simulink model "CLNN_exp_3dof_2NN_exp"  (R2024b)
settings: Solver=ode1  StartTime=0.0  StopTime=T_all  FixedStep=T_sample  RelTol=1e-3
values from neighbouring files (symbols this model uses):
  a1 = m1 * lc1^2 + I1 + (m2 + m3) * l1^2    [plant_robot_3DoF_2NN.m]    (also in setting_3dof_2NN.m = 8.9995)
  a2 = I2 + m2 * lc2^2 + m3 * l2^2    [plant_robot_3DoF_2NN.m]    (also in setting_3dof_2NN.m = 8.9989)
  cl_tf = 300    [run_CLNN_3dof_2NN.m]
  cl_tf1 = 0    [run_CLNN_3dof_2NN.m]
  cl_tf2 = 1050    [run_CLNN_3dof_2NN.m]
  hidden_neure_count_q = 50    [run_CLNN_3dof_2NN.m]
  hidden_neure_count_s = 30    [run_CLNN_3dof_2NN.m]
  kq1 = 0.0026    [setting_3dof_2NN.m]
  kq2 = 0.0011    [setting_3dof_2NN.m]
  lamda = 5    [run_CLNN_3dof_2NN.m]
  lamda_cl = 0.2    [run_CLNN_3dof_2NN.m]
  lamda_cl_s = 0.2    [run_CLNN_3dof_2NN.m]
  learn_time = 100    [run_CLNN_3dof_2NN.m]
  M = [0.001 0 0 ... (first row only)    [run_CLNN_3dof_2NN.m]
  N = 3    [setting_3dof_2NN.m]
  output_dimension_q = 1*N    [run_CLNN_3dof_2NN.m]
  output_dimension_s = 1*N    [run_CLNN_3dof_2NN.m]
  qd20 = 0    [run_CLNN_3dof_2NN.m]
  use_Tqr = 0    [run_CLNN_3dof_2NN.m]
libraries: qbmove_library x3, QB_pacer_lib x1
settings Model: Creator=zou'zhi'gang  LastModifiedBy=zouzgang
settings SolverCC: AlgebraicLoopSolver=TrustRegion
settings DebuggingCC: UnconnectedInputMsg=warning  UnconnectedOutputMsg=warning  UnconnectedLineMsg=warning
settings ModelReferenceCC: EnableRefExpFcnMdlSchedulingChecks=on
settings RTWCC: GPUComputeCapability=3.5

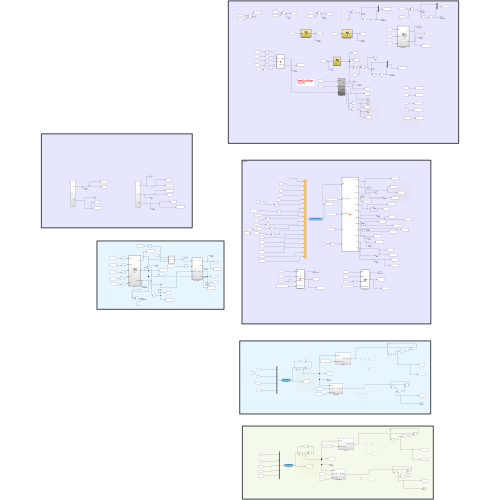
[thumbnail: Simulink's stored preview of the top-level diagram]
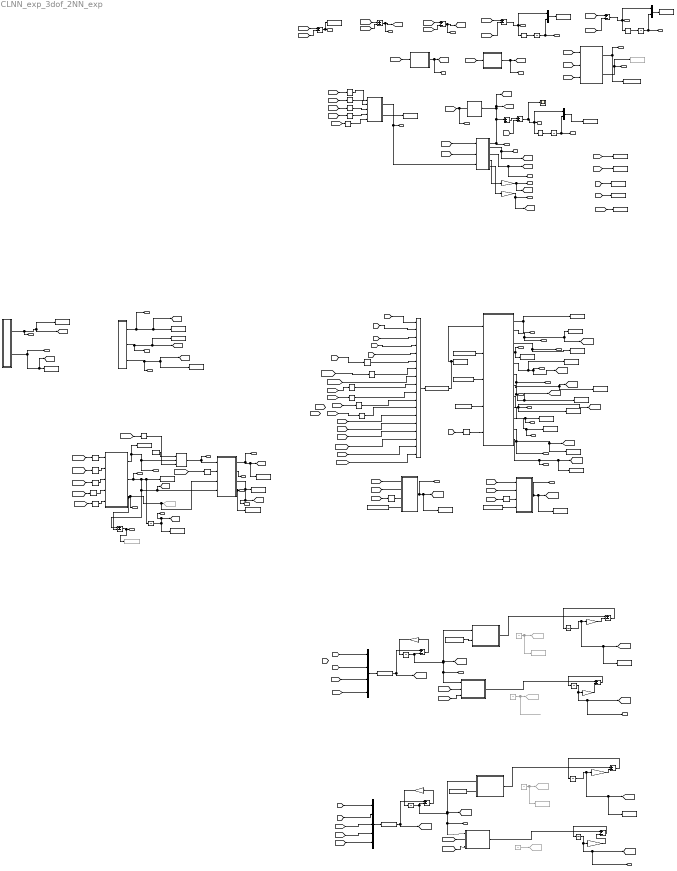
== system CLNN_exp_3dof_2NN_exp ==
  note: 观测器误差
  note: Remember to change the qbmoves IDs and the handle
  Abs1 : Abs  SaturateOnIntegerOverflow=off
  Abs2 : Abs  SaturateOnIntegerOverflow=off
  Abs3 : Abs  SaturateOnIntegerOverflow=off
  Add12 : Sum
  Constant11 : Constant  Value=hidden_neure_count_s
  Constant14 : Constant  Value=N
  Constant16 : Constant  Value=M
  Constant2 : Constant  Value=hidden_neure_count_q
  Constant3 : Constant  Value=hidden_neure_count_s
  Constant4 : Constant  Value=hidden_neure_count_s
  Constant5 : Constant  Value=hidden_neure_count_q
  Constant7 : Constant  Value=hidden_neure_count_q
  Delay{1..21} (21 alike) : Delay  DelayLength=1  InitialCondition=0
  Gain : Gain  Gain=1/265.37
  Gain1 : Gain  Gain=lamda_cl_s
  Gain10 : Gain  Gain=lamda_cl_s
  Gain11 : Gain  Gain=lamda
  Gain12 : Gain  Gain=1/265.37
  Gain2 : Gain  Gain=lamda_cl
  Gain3 : Gain  Gain=lamda_cl
  Gain7 : Gain  Gain=lamda
  Goto3 : Goto  Commented=on  GotoTag=Theta_s
  Goto33 : Goto  Commented=on  GotoTag=Theta_q
  Goto35 : Goto  Commented=on  GotoTag=Theta_W_q
  Goto4 : Goto  Commented=on  GotoTag=Theta_W_s
  Goto83 : Goto  Commented=on  GotoTag=stiff_normal
  Integrator{5..7,12} (4 alike) : Integrator  Commented=on
  Integrator{4,8..9,13..15,17..20} (10 alike) : Integrator
  MATLAB Function : MATLAB Function  TreatAsAtomicUnit=on
  MATLAB Function5 : MATLAB Function  TreatAsAtomicUnit=on
  MATLAB Function6 : MATLAB Function  TreatAsAtomicUnit=on
  Mux1 : Mux  Inputs=[N N N N N]
  Mux2 : Mux  Inputs=[N N N N]
  Mux3 : Mux  Inputs=[N N]
  Mux5 : Mux  Inputs=[N N N N N N N N N N N N N N (hidden_neure_count_q + 1) (hidden_neure_count_q + 1)*output_dimension_q (hidden_neure_count_s + 1) (hidden_neure_count_s + 1)*output_dimension_s]
  Mux7 : Mux  Inputs=[N N]
  Mux8 : Mux  Inputs=[N N]
  Robot : Subsystem
  S-Function4 : S-Function  FunctionName=clnn_control_3dof_2NN  SFunctionDeploymentMode=off  EnableBusSupport=off
  Subsystem4 : Subsystem
  Subtract{1,3..4,6,8,10,14,16..20,22} (13 alike) : Sum  Inputs=+-
  THeta_WW_q : Subsystem
  THeta_WW_s : Subsystem
  Theta error q : MATLAB Function  TreatAsAtomicUnit=on
  Theta error s : MATLAB Function  TreatAsAtomicUnit=on
  Theta_q : Subsystem
  Theta_s : Subsystem
  To Workspace1 : ToWorkspace  VariableName=qd  SampleTime=-1
      settings: Save2DSignal=2-D array (concatenate along first dimension)
  To Workspace10 : ToWorkspace  VariableName=tau_e  SampleTime=-1
      settings: Save2DSignal=2-D array (concatenate along first dimension)
  To Workspace11 : ToWorkspace  VariableName=dqqd  SampleTime=-1
      settings: Save2DSignal=2-D array (concatenate along first dimension)
  To Workspace12 : ToWorkspace  Commented=on  VariableName=Theta_q  SampleTime=-1
      settings: Save2DSignal=2-D array (concatenate along first dimension)
  To Workspace13 : ToWorkspace  VariableName=controlu2  SampleTime=-1
      settings: Save2DSignal=2-D array (concatenate along first dimension)
  To Workspace14 : ToWorkspace  VariableName=controlu1  SampleTime=-1
      settings: Save2DSignal=2-D array (concatenate along first dimension)
  To Workspace15 : ToWorkspace  VariableName=hat_W_q  SampleTime=-1
      settings: Save2DSignal=2-D array (concatenate along first dimension)
  To Workspace16 : ToWorkspace  VariableName=w_un_q_f  SampleTime=-1
      settings: Save2DSignal=2-D array (concatenate along first dimension)
  To Workspace17 : ToWorkspace  Commented=on  VariableName=stiffness1  SampleTime=-1
      settings: Save2DSignal=2-D array (concatenate along first dimension)
  To Workspace18 : ToWorkspace  VariableName=e_S  SampleTime=-1
      settings: Save2DSignal=2-D array (concatenate along first dimension)
  To Workspace19 : ToWorkspace  VariableName=d  SampleTime=-1
      settings: Save2DSignal=2-D array (concatenate along first dimension)
  To Workspace2 : ToWorkspace  VariableName=dqd  SampleTime=-1
      settings: Save2DSignal=2-D array (concatenate along first dimension)
  To Workspace20 : ToWorkspace  VariableName=u_theta1  SampleTime=-1
      settings: Save2DSignal=2-D array (concatenate along first dimension)
  To Workspace21 : ToWorkspace  VariableName=u_theta2  SampleTime=-1
      settings: Save2DSignal=2-D array (concatenate along first dimension)
  To Workspace22 : ToWorkspace  VariableName=e_stiff  SampleTime=-1
      settings: Save2DSignal=2-D array (concatenate along first dimension)
  To Workspace26 : ToWorkspace  VariableName=pd_u  SampleTime=-1
      settings: Save2DSignal=2-D array (concatenate along first dimension)
  To Workspace27 : ToWorkspace  VariableName=model_u  SampleTime=-1
      settings: Save2DSignal=2-D array (concatenate along first dimension)
  To Workspace28 : ToWorkspace  VariableName=Theta_q  SampleTime=-1
      settings: Save2DSignal=2-D array (concatenate along first dimension)
  To Workspace29 : ToWorkspace  Commented=on  VariableName=Theta_s  SampleTime=-1
      settings: Save2DSignal=2-D array (concatenate along first dimension)
  To Workspace30 : ToWorkspace  VariableName=Theta_s  SampleTime=-1
      settings: Save2DSignal=2-D array (concatenate along first dimension)
  To Workspace31 : ToWorkspace  VariableName=Theta_error_s  SampleTime=-1
      settings: Save2DSignal=2-D array (concatenate along first dimension)
  To Workspace33 : ToWorkspace  VariableName=Theta_error_q  SampleTime=-1
      settings: Save2DSignal=2-D array (concatenate along first dimension)
  To Workspace34 : ToWorkspace  VariableName=w_norm_s  SampleTime=-1
      settings: Save2DSignal=2-D array (concatenate along first dimension)
  To Workspace35 : ToWorkspace  VariableName=hat_W_s  SampleTime=-1
      settings: Save2DSignal=2-D array (concatenate along first dimension)
  To Workspace36 : ToWorkspace  VariableName=dstiff  SampleTime=-1
      settings: Save2DSignal=2-D array (concatenate along first dimension)
  To Workspace37 : ToWorkspace  VariableName=dq  SampleTime=-1
      settings: Save2DSignal=2-D array (concatenate along first dimension)
  To Workspace38 : ToWorkspace  VariableName=torque_e  SampleTime=-1
      settings: Save2DSignal=2-D array (concatenate along first dimension)
  To Workspace39 : ToWorkspace  Commented=on  VariableName=stiff_s_nomaic  SampleTime=-1
      settings: Save2DSignal=2-D array (concatenate along first dimension)
  To Workspace4 : ToWorkspace  VariableName=W_V  SampleTime=-1
      settings: Save2DSignal=2-D array (concatenate along first dimension)
  To Workspace40 : ToWorkspace  VariableName=sd  SampleTime=-1
      settings: Save2DSignal=2-D array (concatenate along first dimension)
  To Workspace41 : ToWorkspace  VariableName=stiffness  SampleTime=-1
      settings: Save2DSignal=2-D array (concatenate along first dimension)
  To Workspace42 : ToWorkspace  VariableName=dsd  SampleTime=-1
      settings: Save2DSignal=2-D array (concatenate along first dimension)
  To Workspace43 : ToWorkspace  VariableName=S  SampleTime=-1
      settings: Save2DSignal=2-D array (concatenate along first dimension)
  To Workspace44 : ToWorkspace  VariableName=w_un_s_f  SampleTime=-1
      settings: Save2DSignal=2-D array (concatenate along first dimension)
  To Workspace45 : ToWorkspace  VariableName=tau_e_nomal  SampleTime=-1
      settings: Save2DSignal=2-D array (concatenate along first dimension)
  To Workspace46 : ToWorkspace  VariableName=theta1  SampleTime=-1
      settings: Save2DSignal=2-D array (concatenate along first dimension)
  To Workspace47 : ToWorkspace  VariableName=theta2  SampleTime=-1
      settings: Save2DSignal=2-D array (concatenate along first dimension)
  To Workspace48 : ToWorkspace  VariableName=activation_vec  SampleTime=-1
      settings: Save2DSignal=2-D array (concatenate along first dimension)
  To Workspace49 : ToWorkspace  VariableName=e  SampleTime=-1
      settings: Save2DSignal=2-D array (concatenate along first dimension)
  To Workspace5 : ToWorkspace  VariableName=q  SampleTime=-1
      settings: Save2DSignal=2-D array (concatenate along first dimension)
  To Workspace6 : ToWorkspace  VariableName=w_norm_q  SampleTime=-1
      settings: Save2DSignal=2-D array (concatenate along first dimension)
  To Workspace8 : ToWorkspace  VariableName=epsion  SampleTime=-1
      settings: Save2DSignal=2-D array (concatenate along first dimension)
  To Workspace9 : ToWorkspace  VariableName=w_un_hat  SampleTime=-1
      settings: Save2DSignal=2-D array (concatenate along first dimension)
  Velocity Estimation3 : Subsystem
  Velocity Estimation4 : Subsystem
  Velocity Estimation5 : Subsystem
  phi_3dof_2NN_q : S-Function  FunctionName=phi_3dof_2NN_q  SFunctionDeploymentMode=off  EnableBusSupport=off
  phi_3dof_2NN_s : S-Function  FunctionName=phi_3dof_2NN_s  SFunctionDeploymentMode=off  EnableBusSupport=off
  q-qd : Scope
  s : Subsystem
  stiff and tau1 : Subsystem
  w_un : Subsystem
  w_un_filter : Subsystem  TreatAsAtomicUnit=on
  qd : Outport
  w_un_hat : Outport  Port=2
  WV_q : Outport  Port=3
  epsion : Outport  Port=4
  w_norm : Outport  Port=5
  Theta_error_qq : Outport  Port=6
  controlu1 : Outport  Port=7
  dqd : Outport  Port=8
  dqqd : Outport  Port=9
  tau_e : Outport  Port=10
  w_un_q_f : Outport  Port=11
  phi_filter_q : Outport  Port=12
  controlu2 : Outport  Port=13
  dqq_fq : Outport  Port=14
  u_theta1 : Outport  Port=15
  u_theta2 : Outport  Port=16
  w_q : Outport  Port=17
  model_u : Outport  Port=18
  pd_u : Outport  Port=19
  Theta_W_q : Outport  Port=20
  sd : Outport  Port=21
  dsd : Outport  Port=22
  phi_filter_s : Outport  Port=23
  Theta_W_s : Outport  Port=24
  Theta_error_ss : Outport  Port=25
  w_norm_s : Outport  Port=26
  WV_s : Outport  Port=27
  stiff : Outport  Port=28
  dstiff_nomal : Outport  Port=29
  stiff_s_nomalc : Outport  Port=30
  S : Outport  Port=31
  dS : Outport  Port=32
  w_un_s_f : Outport  Port=33
  dphi1 : Outport  Port=34
  dphi2 : Outport  Port=35
  stiffness1 : Outport  Port=36
  tau_e_nomal1 : Outport  Port=37
  dtheta1 : Outport  Port=38
  dtheta2 : Outport  Port=39
  e : Outport  Port=40
  qe-Integrator : Outport  Port=41
  thtea1 : Outport  Port=42
  theta2 : Outport  Port=43
  q1 : Outport  Port=44
  dq : Outport  Port=45
  activation : Outport  Port=46
  tau1 : Outport  Port=47
  tau2 : Outport  Port=48
  e_S : Outport  Port=49
  e_S-Integrator : Outport  Port=50
  d : Outport  Port=51
  e_stiffness : Outport  Port=52
  e_stiff-Integrator1 : Outport  Port=53
  wires:
  Mux5/1 -> S-Function4/1
  [qd] -> Mux5/1
  [dqd] -> Mux5/2
  [dqqd] -> Mux5/3
  S-Function4/1 -> MATLAB Function6/1(output), To Workspace4/1
  MATLAB Function6/11(W_q) -> WV_q/1, To Workspace15/1, [hat_W_q]
  MATLAB Function6/2(epsion) -> epsion/1, [epsion], To Workspace8/1
  MATLAB Function6/3(w_norm_q) -> To Workspace6/1, w_norm/1
  Integrator6/1 -> To Workspace12/1, Goto33/1
  Integrator7/1 -> Goto35/1
  Integrator8/1 -> Subtract8/2, Theta_q/1(phi_filtter_q), [phi_filter_q], phi_filter_q/1, THeta_WW_q/1(phi_filter)
  Subtract8/1 -> Gain7/1
  Gain7/1 -> Integrator8/1
  [controlu1] -> Mux2/3
  [q] -> Mux2/1
  [controlu2] -> Mux2/4
  Mux2/1 -> phi_3dof_2NN_q/1
  phi_3dof_2NN_q/1 -> [phi_q], Subtract8/1
  [Theta_W_q] -> Theta error q/2(Theta_W_q)
  [Theta_q] -> Theta error q/1(Theta_q)
  Constant7/1 -> Theta error q/4(hidden_neure_count_q)
  Constant5/1 -> Theta_q/2(hidden_neure_count)
  [w_un_q_f] -> THeta_WW_q/2(w_un_q_filter)
  Theta error q/1(Theta_error_q) -> Theta_error_qq/1, To Workspace33/1, [Theta_error_q]
  Constant2/1 -> MATLAB Function6/2(hidden_neure_count_q)
  MATLAB Function6/5(controlu1) -> [controlu1], controlu1/1, To Workspace14/1
  [controlu1] -> Delay1/1
  [controlu2] -> Delay2/1
  Constant14/1 -> MATLAB Function6/4(N)
  MATLAB Function6/1(w_un_hat) -> w_un_hat/1, To Workspace9/1
  Subsystem4/1(qd) -> [qd], To Workspace1/1, qd/1
  Subsystem4/2(dqd) -> To Workspace2/1, [dqd], dqd/1
  Subsystem4/3(dqqd) -> [dqqd], To Workspace11/1, dqqd/1
  w_un/1(tau_e) -> To Workspace10/1, tau_e/1, MATLAB Function/2(tau_e)
  w_un_filter/1(w_un_q_f) -> To Workspace16/1, [w_un_q_f], w_un_q_f/1
  MATLAB Function/1(w_q) -> w_un_filter/1(w_q), w_q/1
  Constant16/1 -> MATLAB Function/1(M)
  MATLAB Function6/6(controlu2) -> To Workspace13/1, [controlu2], controlu2/1
  Delay5/1 -> Theta error q/3(hat_W_vector_q)
  [hat_W_q] -> Delay5/1
  [controlu1] -> Delay6/1
  Delay6/1 -> w_un/1(control_u1)
  [controlu2] -> Delay7/1
  Delay7/1 -> w_un/2(control_u2)
  MATLAB Function6/7(u_theta1) -> u_theta1/1, [u_theta1], To Workspace20/1
  MATLAB Function6/8(u_theta2) -> To Workspace21/1, [u_theta2], u_theta2/1
  [q] -> Delay8/1
  Delay8/1 -> w_un/3(q)
  [q] -> Delay9/1
  [q] -> Delay10/1
  Delay10/1 -> MATLAB Function6/5(q)
  [q] -> Delay12/1
  Delay12/1 -> MATLAB Function/3(q)
  MATLAB Function6/9(pd_u) -> pd_u/1, To Workspace26/1
  MATLAB Function6/10(model_u) -> model_u/1, To Workspace27/1
  Integrator9/1 -> Theta_W_q/1, [Theta_W_q], Gain2/1
  Subtract20/1 -> Integrator15/1
  [dq] -> Mux2/2
  [dq] -> Delay11/1
  THeta_WW_q/1(phi_filter_W_q) -> Subtract10/1
  Gain3/1 -> Subtract20/2
  Integrator15/1 -> Gain3/1, [Theta_q], To Workspace28/1
  Subtract10/1 -> Integrator9/1
  Gain2/1 -> Subtract10/2
  [dq] -> Delay4/1
  Delay11/1 -> w_un_filter/2(dq)
  s/2(Sd) -> sd/1, To Workspace40/1, [sd]
  s/1(dsd) -> dsd/1, To Workspace42/1, [dsd]
  w_un/2(stiff) -> stiff/1, Integrator18/1, To Workspace41/1, [stiffness], w_un_filter/4(stiff), Subtract16/1
  w_un/3(stiff_normal) -> w_un_filter/3(stiff_normal), Goto83/1, dstiff_nomal/1, Subtract16/2
  w_un_filter/2(dqq) -> dqq_fq/1
  w_un_filter/3(w_un_s_f) -> w_un_s_f/1, [w_un_s_f], To Workspace44/1
  [w_un_s_f] -> THeta_WW_q/3(w_un_s_filter)
  Delay1/1 -> Mux5/9
  Delay2/1 -> Mux5/10
  [S] -> Mux5/8
  Delay4/1 -> Mux5/7
  Delay9/1 -> Mux5/6
  [sd] -> Mux5/4
  [dsd] -> Mux5/5
  [w_un_q_f] -> THeta_WW_s/2(w_un_q_filter)
  phi_3dof_2NN_s/1 -> [phi_s], Subtract4/1
  Mux1/1 -> phi_3dof_2NN_s/1
  Gain11/1 -> Integrator13/1
  Integrator12/1 -> Goto4/1
  Constant3/1 -> Theta_s/2(hidden_neure_count)
  [dphi1] -> Mux1/1
  Subtract3/1 -> Integrator4/1
  Integrator14/1 -> Theta_W_s/1, [Theta_W_s], Gain1/1
  Gain10/1 -> Subtract3/2
  [controlu1] -> Mux1/3
  Integrator4/1 -> Gain10/1, [Theta_s], To Workspace30/1
  [w_un_s_f] -> THeta_WW_s/3(w_un_s_filter)
  [dphi2] -> Mux1/2
  [controlu2] -> Mux1/4
  Subtract4/1 -> Gain11/1
  Subtract1/1 -> Integrator14/1
  Integrator13/1 -> Subtract4/2, Theta_s/1(phi_filtter_s), [phi_filter_s], phi_filter_s/1, THeta_WW_s/1(phi_filter)
  Integrator5/1 -> To Workspace29/1, Goto3/1
  Gain1/1 -> Subtract1/2
  Theta error s/1(Theta_error_s) -> Theta_error_ss/1, To Workspace31/1, [Theta_error_s]
  Constant4/1 -> Theta error s/4(hidden_neure_count_s)
  [Theta_s] -> Theta error s/1(Theta_s)
  [Theta_W_s] -> Theta error s/2(Theta_W_s)
  Delay13/1 -> Theta error s/3(hat_W_vector_s)
  [hat_W_s] -> Delay13/1
  Constant11/1 -> MATLAB Function6/3(hidden_neure_count_s)
  MATLAB Function6/4(w_norm_s) -> To Workspace34/1, w_norm_s/1
  MATLAB Function6/12(W_s) -> WV_s/1, To Workspace35/1, [hat_W_s]
  [theta1] -> Delay14/1
  Delay14/1 -> w_un/4(theta1)
  Delay15/1 -> w_un/5(theta2)
  [theta2] -> Delay15/1
  Subtract16/1 -> To Workspace39/1, stiff_s_nomalc/1
  [w_un_q_f] -> Mux5/13
  [w_un_s_f] -> Mux5/14
  [phi_filter_q] -> Mux5/15
  [Theta_error_q] -> Mux5/16
  [phi_filter_s] -> Mux5/17
  [Theta_error_s] -> Mux5/18
  [dtheta1] -> Delay16/1
  [dtheta2] -> Delay17/1
  Delay17/1 -> Mux5/12
  Delay16/1 -> Mux5/11
  w_un_filter/4(dS) -> To Workspace36/1, dS/1
  [dq] -> Mux1/5
  Integrator18/1 -> To Workspace43/1, S/1, [S]
  [q] -> stiff and tau1/3(q)
  [theta1] -> Delay18/1
  [dq] -> To Workspace37/1
  Robot/2(theta1) -> [theta1], thtea1/1
  [q] -> To Workspace5/1
  [torque_e] -> To Workspace38/1
  Velocity Estimation3/1(dtheta1) -> dtheta1/1, [dtheta1]
  stiff and tau1/2(stiff) -> To Workspace17/1, stiffness1/1
  MATLAB Function5/1(activation) -> activation/1, Robot/3(activation)
  Robot/3(theta2) -> theta2/1, [theta2]
  [theta2] -> Delay19/1
  [dtheta2] -> Subtract18/2
  [theta2] -> To Workspace47/1
  Gain/1 -> [tau1], tau1/1
  Gain12/1 -> [tau2], tau2/1
  stiff and tau1/1(tau_e) -> tau_e_nomal1/1, To Workspace45/1
  Robot/1(q) -> q1/1, Velocity Estimation5/1(q), [q], [q_inner], Add12/1
  Subtract14/1 -> q-qd/1, Mux3/1, e/1, Abs1/1
  [theta2] -> stiff and tau1/2(theta2)
  [theta1] -> To Workspace46/1
  [dq] -> Subtract17/1
  Integrator17/1 -> Mux3/2, qe-Integrator/1
  Delay18/1 -> MATLAB Function5/2(theta1)
  Mux3/1 -> To Workspace49/1
  Velocity Estimation4/1(dtheta2) -> dtheta2/1, [dtheta2]
  Robot/4(current1) -> Gain/1
  Delay3/1 -> MATLAB Function5/1(q)
  [theta1] -> stiff and tau1/1(theta1)
  [qd] -> Subtract14/2
  Add12/1 -> Subtract14/1
  [theta2] -> Velocity Estimation4/1(theta2)
  [theta1] -> Velocity Estimation3/1(theta1)
  [dtheta1] -> Subtract17/2
  Delay19/1 -> MATLAB Function5/3(theta2)
  Velocity Estimation5/1(dq) -> dq/1, [dq]
  Robot/5(current2) -> Gain12/1
  Abs1/1 -> Integrator17/1
  [dq] -> Subtract18/1
  [q] -> Delay3/1
  MATLAB Function5/2(activation_vec) -> To Workspace48/1
  Subtract17/1 -> [dphi1], dphi1/1
  Subtract18/1 -> [dphi2], dphi2/1
  Mux7/1 -> To Workspace18/1
  [sd] -> Subtract19/1
  Abs2/1 -> Integrator19/1
  [S] -> Subtract19/2
  Subtract19/1 -> Mux7/1, e_S/1, Abs2/1
  Integrator19/1 -> Mux7/2, e_S-Integrator/1
  [theta2] -> Subtract22/2
  [theta1] -> Subtract22/1
  Subtract22/1 -> To Workspace19/1, d/1
  Subtract6/1 -> Mux8/1, e_stiffness/1, Abs3/1
  [stiffness] -> Subtract6/2
  Integrator20/1 -> Mux8/2, e_stiff-Integrator1/1
  [dsd] -> Subtract6/1
  Abs3/1 -> Integrator20/1
  Mux8/1 -> To Workspace22/1
  Theta_q/1(phi_filter_phi_filte_q) -> Subtract20/1
  Theta_s/1(phi_filter_phi_filter) -> Subtract3/1
  THeta_WW_s/1(phi_filter_W_s) -> Subtract1/1
  [u_theta2] -> Robot/2(u_theta2)
  [u_theta1] -> Robot/1(u_theta1)
  Delay20/1 -> MATLAB Function5/4(u1)
  [u_theta1] -> Delay20/1
  [u_theta2] -> Delay21/1
  Delay21/1 -> MATLAB Function5/5(u2)

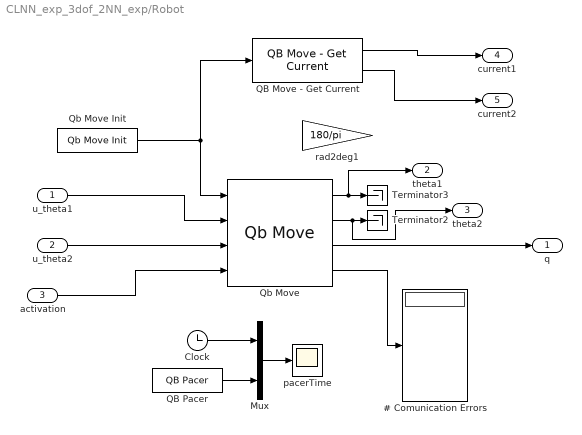
== system CLNN_exp_3dof_2NN_exp/Robot ==
  u_theta1 : Inport
  u_theta2 : Inport  Port=2
  activation : Inport  Port=3
  # Comunication Errors : Display
  Clock : Clock
  Mux : Mux  Inputs=2
  QB Move - Get Current : qbmove_library/QB Move - Get Current  ID=[1,2,3]  CONTROL_MODE=Prime Movers Positions  DAISY_CHAINING=off
      settings: SourceProductName=Qb Move Library
  QB Pacer : QB_pacer_lib/QB Pacer  simTimePerRealTime=1
      settings: SourceProductName=QB Pacer
  Qb Move : qbmove_library/Qb Move  ID=[1,2,3]  ACTIVE_COMM_DIRECTIONS=Both  CONTROL_MODE=Prime Movers Positions  DAISY_CHAINING=off  MAX_ANG=0  SW_LIMIT=inf  OFFSET=0  ACTIVATE=off  WDT=0.0  UNIT=Radians
      settings: SourceProductName=Qb Move Library
  Qb Move Init : qbmove_library/Qb Move Init  NUMBER_OF_COM='COM19'  BAUD_RATE_COM=2000000
      settings: SourceProductName=Qb Move Library
  Terminator2 : Terminator
  Terminator3 : Terminator
  pacerTime : Scope
  rad2deg1 : Gain  Gain=180/pi
  q : Outport
  theta1 : Outport  Port=2
  theta2 : Outport  Port=3
  current1 : Outport  Port=4
  current2 : Outport  Port=5
  wires:
  QB Pacer/1 -> Mux/2
  Clock/1 -> Mux/1
  Qb Move Init/1 -> Qb Move/1, QB Move - Get Current/1
  Mux/1 -> pacerTime/1
  Qb Move/1 -> theta1/1, Terminator3/1
  Qb Move/2 -> theta2/1, Terminator2/1
  u_theta1/1 -> Qb Move/2
  Qb Move/4 -> # Comunication Errors/1
  u_theta2/1 -> Qb Move/3
  Qb Move/3 -> q/1
  activation/1 -> Qb Move/4
  QB Move - Get Current/1 -> current1/1
  QB Move - Get Current/2 -> current2/1

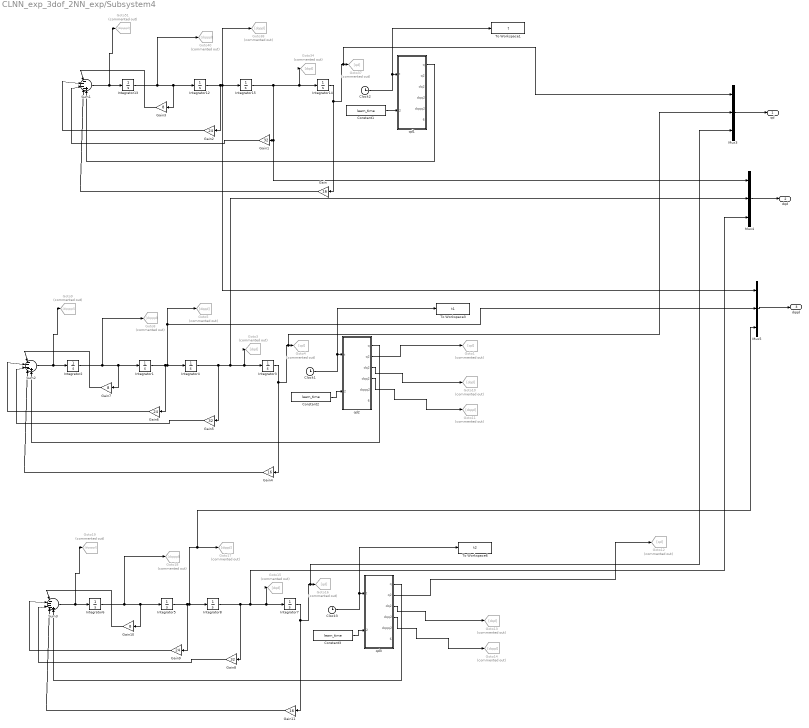
== system CLNN_exp_3dof_2NN_exp/Subsystem4 ==
  Clock1 : Clock
  Clock2 : Clock
  Clock3 : Clock
  Constant1 : Constant  Value=learn_time
  Constant2 : Constant  Value=learn_time
  Constant3 : Constant  Value=learn_time
  Gain : Gain  Gain=16
  Gain1 : Gain  Gain=32
  Gain10 : Gain  Gain=8
  Gain11 : Gain  Gain=16
  Gain2 : Gain  Gain=24
  Gain3 : Gain  Gain=8
  Gain4 : Gain  Gain=16
  Gain5 : Gain  Gain=32
  Gain6 : Gain  Gain=24
  Gain7 : Gain  Gain=8
  Gain8 : Gain  Gain=32
  Gain9 : Gain  Gain=24
  Goto{1,4,12,16,37} (5 alike) : Goto  Commented=on  GotoTag=qd
  Goto{3,10,13,15,34} (5 alike) : Goto  Commented=on  GotoTag=dqd
  Goto{5,11,14,17,38} (5 alike) : Goto  Commented=on  GotoTag=dqqd
  Goto18 : Goto  Commented=on  GotoTag=dqqqd
  Goto19 : Goto  Commented=on  GotoTag=dqqqqd
  Goto40 : Goto  Commented=on  GotoTag=dqqqd
  Goto51 : Goto  Commented=on  GotoTag=dqqqqd
  Goto8 : Goto  Commented=on  GotoTag=dqqqd
  Goto9 : Goto  Commented=on  GotoTag=dqqqqd
  Integrator{1..2,4..8,12..15} (11 alike) : Integrator
  Integrator3 : Integrator  InitialCondition=qd20
  Mux3 : Mux  Inputs=3
  Mux4 : Mux  Inputs=3
  Mux5 : Mux  Inputs=3
  Sum1 : Sum  Inputs=|----+
  Sum2 : Sum  Inputs=|----+
  Sum3 : Sum  Inputs=|----+
  To Workspace1 : ToWorkspace  VariableName=t  SaveFormat=Timeseries  SampleTime=-1
  To Workspace3 : ToWorkspace  VariableName=t1  SaveFormat=Timeseries  SampleTime=-1
  To Workspace6 : ToWorkspace  VariableName=t2  SaveFormat=Timeseries  SampleTime=-1
  qd1 : MATLAB Function  TreatAsAtomicUnit=on
  qd2 : MATLAB Function  TreatAsAtomicUnit=on
  qd3 : MATLAB Function  TreatAsAtomicUnit=on
  qd : Outport
  dqd : Outport  Port=2
  dqqd : Outport  Port=3
  wires:
  Clock2/1 -> To Workspace1/1, qd1/1(t)
  Integrator15/1 -> Mux4/1, Gain1/1, Goto34/1, Integrator14/1
  Integrator13/1 -> Goto40/1, Gain3/1, Integrator12/1
  Sum1/1 -> Goto51/1, Integrator13/1
  Integrator14/1 -> Mux3/1, Goto37/1, Gain/1
  Gain/1 -> Sum1/4
  Integrator12/1 -> Gain2/1, Mux5/1, Goto38/1, Integrator15/1
  Gain2/1 -> Sum1/2
  Gain3/1 -> Sum1/1
  Gain1/1 -> Sum1/3
  qd1/1(q) -> Sum1/5
  Gain5/1 -> Sum2/3
  qd2/1(q) -> Sum2/5
  Gain6/1 -> Sum2/2
  qd2/3(dq2) -> Goto10/1
  Gain7/1 -> Sum2/1
  Integrator1/1 -> Gain6/1, Mux5/2, Goto5/1, Integrator4/1
  qd2/2(q2) -> Goto1/1
  Integrator3/1 -> Mux3/2, Goto4/1, Gain4/1
  qd2/4(dqq2) -> Goto11/1
  Integrator2/1 -> Goto8/1, Gain7/1, Integrator1/1
  Sum2/1 -> Goto9/1, Integrator2/1
  Gain4/1 -> Sum2/4
  Clock1/1 -> To Workspace3/1, qd2/1(t)
  Integrator4/1 -> Gain5/1, Mux4/2, Goto3/1, Integrator3/1
  Integrator7/1 -> Gain11/1, Mux3/3, Goto16/1
  Clock3/1 -> To Workspace6/1, qd3/1(t)
  Integrator8/1 -> Gain8/1, Mux4/3, Goto15/1, Integrator7/1
  Gain10/1 -> Sum3/1
  qd3/2(q2) -> Goto12/1
  qd3/4(dqq2) -> Goto14/1
  Gain8/1 -> Sum3/3
  Sum3/1 -> Goto19/1, Integrator6/1
  Integrator6/1 -> Goto18/1, Gain10/1, Integrator5/1
  Gain9/1 -> Sum3/2
  Gain11/1 -> Sum3/4
  qd3/1(q) -> Sum3/5
  Integrator5/1 -> Gain9/1, Mux5/3, Goto17/1, Integrator8/1
  qd3/3(dq2) -> Goto13/1
  Mux3/1 -> qd/1
  Mux4/1 -> dqd/1
  Mux5/1 -> dqqd/1
  Constant1/1 -> qd1/2(learn_time)
  Constant2/1 -> qd2/2(learn_time)
  Constant3/1 -> qd3/2(learn_time)

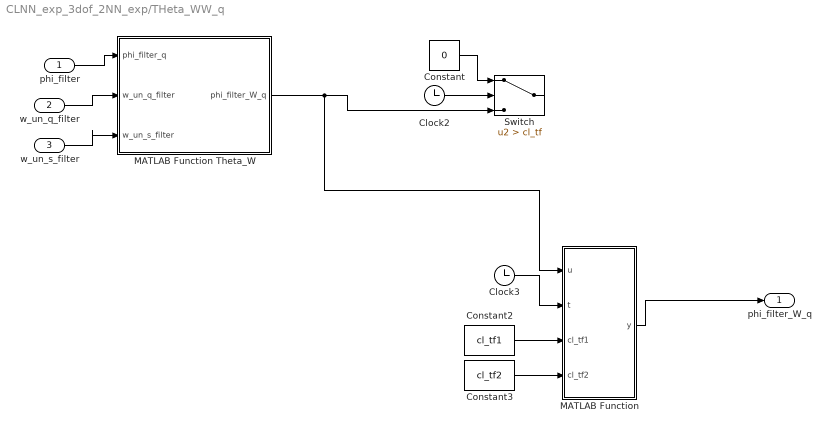
== system CLNN_exp_3dof_2NN_exp/THeta_WW_q ==
  phi_filter : Inport
  w_un_q_filter : Inport  Port=2
  w_un_s_filter : Inport  Port=3
  Clock2 : Clock
  Clock3 : Clock
  Constant : Constant  Value=0
  Constant2 : Constant  Value=cl_tf1
  Constant3 : Constant  Value=cl_tf2
  MATLAB Function : MATLAB Function  TreatAsAtomicUnit=on
  MATLAB Function Theta_W : MATLAB Function  TreatAsAtomicUnit=on
  Switch : Switch  Criteria=u2 > Threshold  Threshold=cl_tf  SaturateOnIntegerOverflow=off  InputSameDT=off
  phi_filter_W_q : Outport
  wires:
  w_un_q_filter/1 -> MATLAB Function Theta_W/2(w_un_q_filter)
  phi_filter/1 -> MATLAB Function Theta_W/1(phi_filter_q)
  Clock2/1 -> Switch/2
  Constant/1 -> Switch/1
  MATLAB Function/1(y) -> phi_filter_W_q/1
  Constant3/1 -> MATLAB Function/4(cl_tf2)
  Clock3/1 -> MATLAB Function/2(t)
  Constant2/1 -> MATLAB Function/3(cl_tf1)
  MATLAB Function Theta_W/1(phi_filter_W_q) -> MATLAB Function/1(u), Switch/3
  w_un_s_filter/1 -> MATLAB Function Theta_W/3(w_un_s_filter)

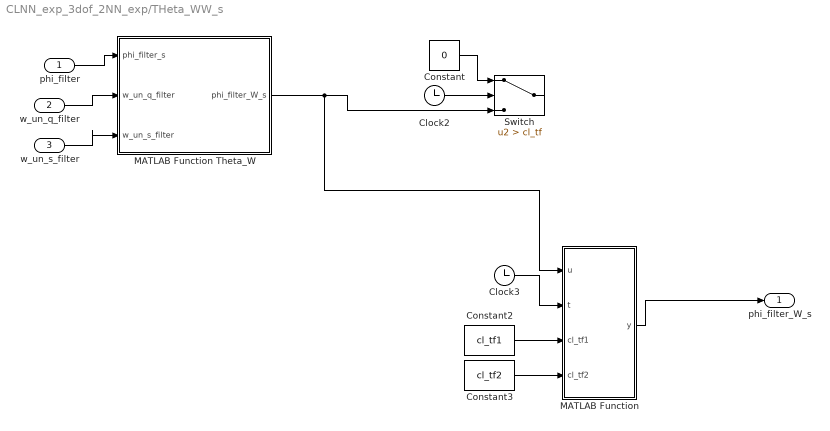
== system CLNN_exp_3dof_2NN_exp/THeta_WW_s ==
  phi_filter : Inport
  w_un_q_filter : Inport  Port=2
  w_un_s_filter : Inport  Port=3
  Clock2 : Clock
  Clock3 : Clock
  Constant : Constant  Value=0
  Constant2 : Constant  Value=cl_tf1
  Constant3 : Constant  Value=cl_tf2
  MATLAB Function : MATLAB Function  TreatAsAtomicUnit=on
  MATLAB Function Theta_W : MATLAB Function  TreatAsAtomicUnit=on
  Switch : Switch  Criteria=u2 > Threshold  Threshold=cl_tf  SaturateOnIntegerOverflow=off  InputSameDT=off
  phi_filter_W_s : Outport
  wires:
  w_un_q_filter/1 -> MATLAB Function Theta_W/2(w_un_q_filter)
  phi_filter/1 -> MATLAB Function Theta_W/1(phi_filter_s)
  Clock2/1 -> Switch/2
  Constant/1 -> Switch/1
  MATLAB Function/1(y) -> phi_filter_W_s/1
  Constant3/1 -> MATLAB Function/4(cl_tf2)
  Clock3/1 -> MATLAB Function/2(t)
  Constant2/1 -> MATLAB Function/3(cl_tf1)
  MATLAB Function Theta_W/1(phi_filter_W_s) -> MATLAB Function/1(u), Switch/3
  w_un_s_filter/1 -> MATLAB Function Theta_W/3(w_un_s_filter)

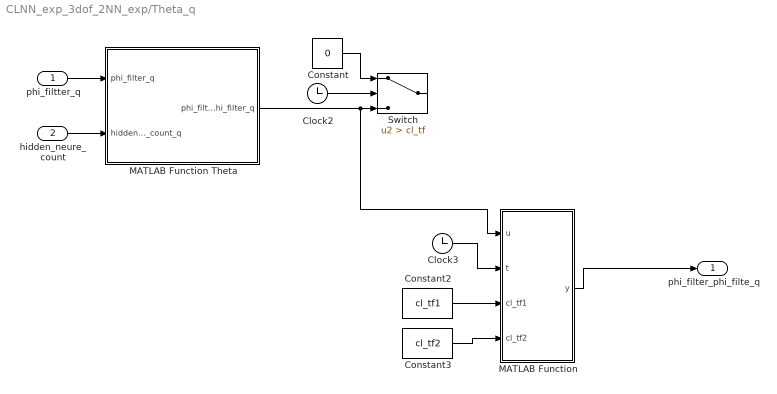
== system CLNN_exp_3dof_2NN_exp/Theta_q ==
  phi_filtter_q : Inport
  hidden_neure_count : Inport  Port=2
  Clock2 : Clock
  Clock3 : Clock
  Constant : Constant  Value=0
  Constant2 : Constant  Value=cl_tf1
  Constant3 : Constant  Value=cl_tf2
  MATLAB Function : MATLAB Function  TreatAsAtomicUnit=on
  MATLAB Function Theta : MATLAB Function  TreatAsAtomicUnit=on
  Switch : Switch  Criteria=u2 > Threshold  Threshold=cl_tf  SaturateOnIntegerOverflow=off  InputSameDT=off
  phi_filter_phi_filte_q : Outport
  wires:
  phi_filtter_q/1 -> MATLAB Function Theta/1(phi_filter_q)
  hidden_neure_count/1 -> MATLAB Function Theta/2(hidden_neure_count_q)
  Clock2/1 -> Switch/2
  Constant/1 -> Switch/1
  MATLAB Function/1(y) -> phi_filter_phi_filte_q/1
  Constant2/1 -> MATLAB Function/3(cl_tf1)
  Constant3/1 -> MATLAB Function/4(cl_tf2)
  MATLAB Function Theta/1(phi_filter_phi_filter_q) -> MATLAB Function/1(u), Switch/3
  Clock3/1 -> MATLAB Function/2(t)

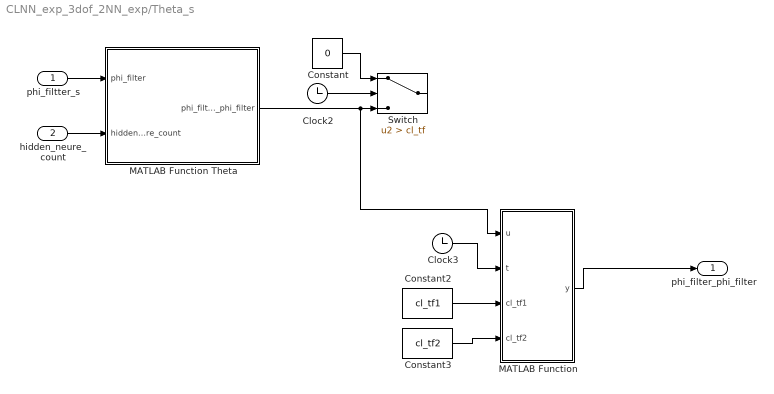
== system CLNN_exp_3dof_2NN_exp/Theta_s ==
  phi_filtter_s : Inport
  hidden_neure_count : Inport  Port=2
  Clock2 : Clock
  Clock3 : Clock
  Constant : Constant  Value=0
  Constant2 : Constant  Value=cl_tf1
  Constant3 : Constant  Value=cl_tf2
  MATLAB Function : MATLAB Function  TreatAsAtomicUnit=on
  MATLAB Function Theta : MATLAB Function  TreatAsAtomicUnit=on
  Switch : Switch  Criteria=u2 > Threshold  Threshold=cl_tf  SaturateOnIntegerOverflow=off  InputSameDT=off
  phi_filter_phi_filter : Outport
  wires:
  phi_filtter_s/1 -> MATLAB Function Theta/1(phi_filter)
  hidden_neure_count/1 -> MATLAB Function Theta/2(hidden_neure_count)
  Clock2/1 -> Switch/2
  Constant/1 -> Switch/1
  MATLAB Function/1(y) -> phi_filter_phi_filter/1
  Constant2/1 -> MATLAB Function/3(cl_tf1)
  Constant3/1 -> MATLAB Function/4(cl_tf2)
  MATLAB Function Theta/1(phi_filter_phi_filter) -> MATLAB Function/1(u), Switch/3
  Clock3/1 -> MATLAB Function/2(t)

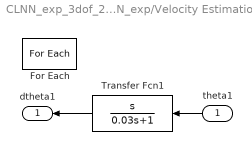
== system CLNN_exp_3dof_2NN_exp/Velocity Estimation3 ==
  theta1 : Inport  Partition=on  PartitionDimension=1  PartitionWidth=1  PartitionOffset=0
  For Each : ForEach  DisableCoverage=on
  Transfer Fcn1 : TransferFcn  Numerator=[1 0]  Denominator=[0.03 1]
  dtheta1 : Outport  ConcatenationDimension=1
  wires:
  theta1/1 -> Transfer Fcn1/1
  Transfer Fcn1/1 -> dtheta1/1

== system CLNN_exp_3dof_2NN_exp/Velocity Estimation4 ==
  theta2 : Inport  Partition=on  PartitionDimension=1  PartitionWidth=1  PartitionOffset=0
  For Each : ForEach  DisableCoverage=on
  Transfer Fcn1 : TransferFcn  Numerator=[1 0]  Denominator=[0.03 1]
  dtheta2 : Outport  ConcatenationDimension=1
  wires:
  theta2/1 -> Transfer Fcn1/1
  Transfer Fcn1/1 -> dtheta2/1

== system CLNN_exp_3dof_2NN_exp/Velocity Estimation5 ==
  q : Inport  Partition=on  PartitionDimension=1  PartitionWidth=1  PartitionOffset=0
  For Each : ForEach  DisableCoverage=on
  Transfer Fcn1 : TransferFcn  Numerator=[1 0]  Denominator=[0.03 1]
  dq : Outport  ConcatenationDimension=1
  wires:
  q/1 -> Transfer Fcn1/1
  Transfer Fcn1/1 -> dq/1

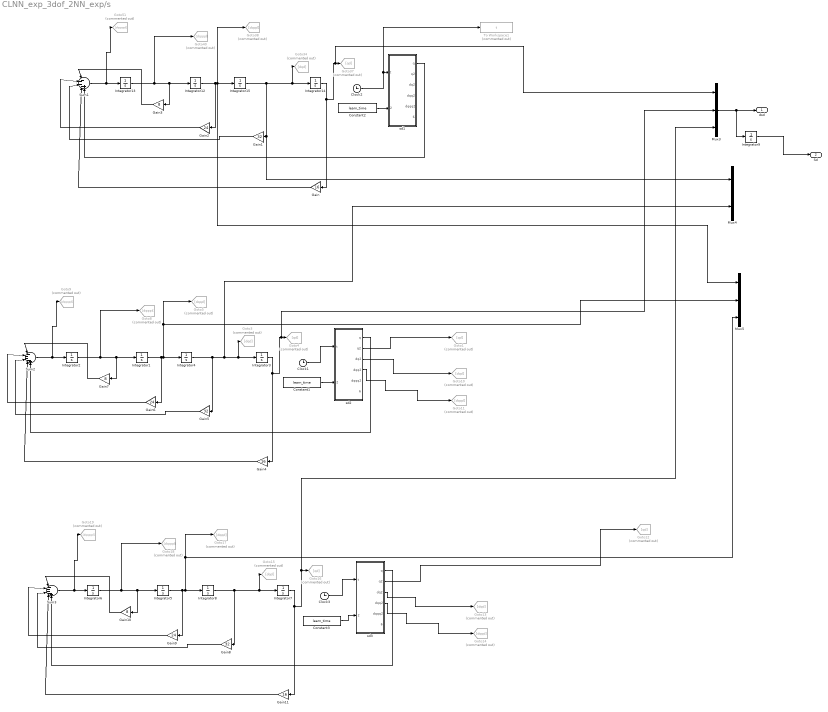
== system CLNN_exp_3dof_2NN_exp/s ==
  Clock1 : Clock
  Clock2 : Clock
  Clock3 : Clock
  Constant1 : Constant  Value=learn_time
  Constant2 : Constant  Value=learn_time
  Constant3 : Constant  Value=learn_time
  Gain : Gain  Gain=16
  Gain1 : Gain  Gain=32
  Gain10 : Gain  Gain=8
  Gain11 : Gain  Gain=16
  Gain2 : Gain  Gain=24
  Gain3 : Gain  Gain=8
  Gain4 : Gain  Gain=16
  Gain5 : Gain  Gain=32
  Gain6 : Gain  Gain=24
  Gain7 : Gain  Gain=8
  Gain8 : Gain  Gain=32
  Gain9 : Gain  Gain=24
  Goto{1,4,12,16,37} (5 alike) : Goto  Commented=on  GotoTag=qd
  Goto{3,10,13,15,34} (5 alike) : Goto  Commented=on  GotoTag=dqd
  Goto{5,11,14,17,38} (5 alike) : Goto  Commented=on  GotoTag=dqqd
  Goto18 : Goto  Commented=on  GotoTag=dqqqd
  Goto19 : Goto  Commented=on  GotoTag=dqqqqd
  Goto40 : Goto  Commented=on  GotoTag=dqqqd
  Goto51 : Goto  Commented=on  GotoTag=dqqqqd
  Goto8 : Goto  Commented=on  GotoTag=dqqqd
  Goto9 : Goto  Commented=on  GotoTag=dqqqqd
  Integrator{1..8,12..13,15} (11 alike) : Integrator
  Integrator14 : Integrator  InitialCondition=0.0333
  Integrator9 : Integrator  InitialCondition=0.0333
  Mux3 : Mux  Inputs=3
  Mux4 : Mux  Inputs=2
  Mux5 : Mux  Inputs=3
  Sum1 : Sum  Inputs=|----+
  Sum2 : Sum  Inputs=|----+
  Sum3 : Sum  Inputs=|----+
  To Workspace1 : ToWorkspace  Commented=on  VariableName=t  SaveFormat=Timeseries  SampleTime=-1
  sd1 : MATLAB Function  TreatAsAtomicUnit=on
  sd2 : MATLAB Function  TreatAsAtomicUnit=on
  sd3 : MATLAB Function  TreatAsAtomicUnit=on
  dsd : Outport
  Sd : Outport  Port=2
  wires:
  Clock2/1 -> To Workspace1/1, sd1/1(t)
  Integrator15/1 -> Mux4/1, Gain1/1, Goto34/1, Integrator14/1
  Integrator13/1 -> Goto40/1, Gain3/1, Integrator12/1
  Sum1/1 -> Goto51/1, Integrator13/1
  Integrator14/1 -> Mux3/1, Goto37/1, Gain/1
  Gain/1 -> Sum1/4
  Integrator12/1 -> Gain2/1, Mux5/1, Goto38/1, Integrator15/1
  Gain2/1 -> Sum1/2
  Gain3/1 -> Sum1/1
  Gain1/1 -> Sum1/3
  sd1/1(q) -> Sum1/5
  Gain5/1 -> Sum2/3
  sd2/1(q) -> Sum2/5
  Gain6/1 -> Sum2/2
  sd2/3(dq2) -> Goto10/1
  Gain7/1 -> Sum2/1
  Integrator1/1 -> Gain6/1, Mux5/2, Goto5/1, Integrator4/1
  sd2/2(q2) -> Goto1/1
  Integrator3/1 -> Mux3/2, Goto4/1, Gain4/1
  sd2/4(dqq2) -> Goto11/1
  Integrator2/1 -> Goto8/1, Gain7/1, Integrator1/1
  Sum2/1 -> Goto9/1, Integrator2/1
  Gain4/1 -> Sum2/4
  Clock1/1 -> sd2/1(t)
  Integrator4/1 -> Gain5/1, Mux4/2, Goto3/1, Integrator3/1
  Integrator7/1 -> Gain11/1, Mux3/3, Goto16/1
  Clock3/1 -> sd3/1(t)
  Integrator8/1 -> Gain8/1, Goto15/1, Integrator7/1
  Gain10/1 -> Sum3/1
  sd3/2(q2) -> Goto12/1
  sd3/4(dqq2) -> Goto14/1
  Gain8/1 -> Sum3/3
  Sum3/1 -> Goto19/1, Integrator6/1
  Integrator6/1 -> Goto18/1, Gain10/1, Integrator5/1
  Gain9/1 -> Sum3/2
  Gain11/1 -> Sum3/4
  sd3/1(q) -> Sum3/5
  Integrator5/1 -> Gain9/1, Mux5/3, Goto17/1, Integrator8/1
  sd3/3(dq2) -> Goto13/1
  Mux3/1 -> Integrator9/1, dsd/1
  Integrator9/1 -> Sd/1
  Constant2/1 -> sd1/2(learn_time)
  Constant1/1 -> sd2/2(learn_time)
  Constant3/1 -> sd3/2(learn_time)

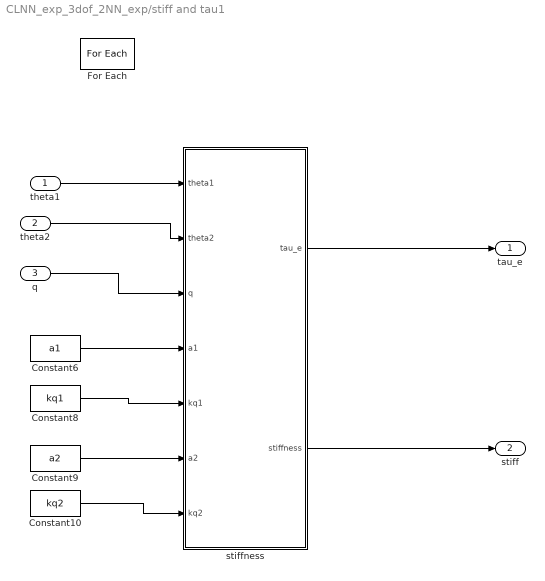
== system CLNN_exp_3dof_2NN_exp/stiff and tau1 ==
  theta1 : Inport  Partition=on  PartitionDimension=1  PartitionWidth=1  PartitionOffset=0
  theta2 : Inport  Port=2  Partition=on  PartitionDimension=1  PartitionWidth=1  PartitionOffset=0
  q : Inport  Port=3  Partition=on  PartitionDimension=1  PartitionWidth=1  PartitionOffset=0
  Constant10 : Constant  Value=kq2
  Constant6 : Constant  Value=a1
  Constant8 : Constant  Value=kq1
  Constant9 : Constant  Value=a2
  For Each : ForEach  DisableCoverage=on
  stiffness : MATLAB Function  TreatAsAtomicUnit=on
  tau_e : Outport  ConcatenationDimension=1
  stiff : Outport  Port=2  ConcatenationDimension=1
  wires:
  theta2/1 -> stiffness/2(theta2)
  stiffness/1(tau_e) -> tau_e/1
  theta1/1 -> stiffness/1(theta1)
  Constant6/1 -> stiffness/4(a1)
  Constant8/1 -> stiffness/5(kq1)
  Constant9/1 -> stiffness/6(a2)
  Constant10/1 -> stiffness/7(kq2)
  q/1 -> stiffness/3(q)
  stiffness/2(stiffness) -> stiff/1

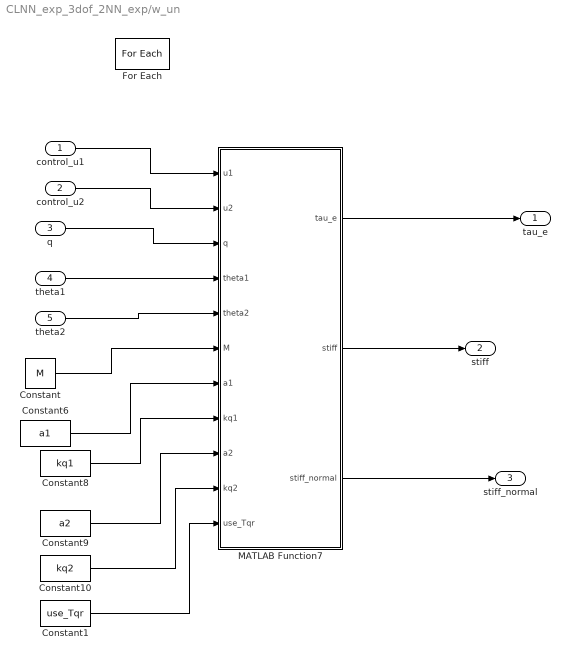
== system CLNN_exp_3dof_2NN_exp/w_un ==
  control_u1 : Inport  Partition=on  PartitionDimension=1  PartitionWidth=1  PartitionOffset=0
  control_u2 : Inport  Port=2  Partition=on  PartitionDimension=1  PartitionWidth=1  PartitionOffset=0
  q : Inport  Port=3  Partition=on  PartitionDimension=1  PartitionWidth=1  PartitionOffset=0
  theta1 : Inport  Port=4  Partition=on  PartitionDimension=1  PartitionWidth=1  PartitionOffset=0
  theta2 : Inport  Port=5  Partition=on  PartitionDimension=1  PartitionWidth=1  PartitionOffset=0
  Constant : Constant  Value=M
  Constant1 : Constant  Value=use_Tqr
  Constant10 : Constant  Value=kq2
  Constant6 : Constant  Value=a1
  Constant8 : Constant  Value=kq1
  Constant9 : Constant  Value=a2
  For Each : ForEach  DisableCoverage=on
  MATLAB Function7 : MATLAB Function  TreatAsAtomicUnit=on
  tau_e : Outport  ConcatenationDimension=1
  stiff : Outport  Port=2  ConcatenationDimension=1
  stiff_normal : Outport  Port=3  ConcatenationDimension=1
  wires:
  control_u2/1 -> MATLAB Function7/2(u2)
  MATLAB Function7/1(tau_e) -> tau_e/1
  control_u1/1 -> MATLAB Function7/1(u1)
  Constant6/1 -> MATLAB Function7/7(a1)
  Constant8/1 -> MATLAB Function7/8(kq1)
  Constant9/1 -> MATLAB Function7/9(a2)
  Constant10/1 -> MATLAB Function7/10(kq2)
  Constant/1 -> MATLAB Function7/6(M)
  q/1 -> MATLAB Function7/3(q)
  Constant1/1 -> MATLAB Function7/11(use_Tqr)
  MATLAB Function7/3(stiff_normal) -> stiff_normal/1
  MATLAB Function7/2(stiff) -> stiff/1
  theta1/1 -> MATLAB Function7/4(theta1)
  theta2/1 -> MATLAB Function7/5(theta2)

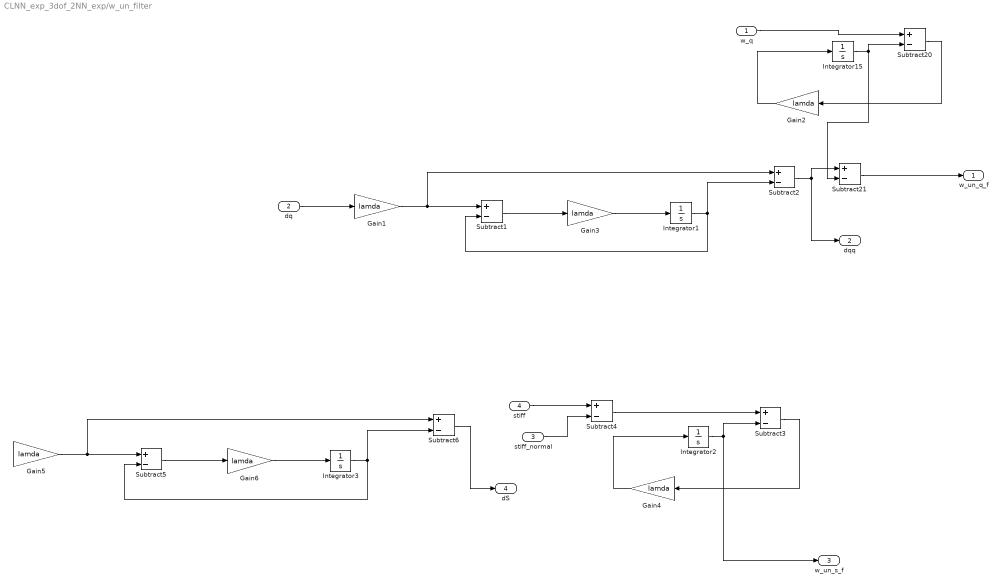
== system CLNN_exp_3dof_2NN_exp/w_un_filter ==
  w_q : Inport
  dq : Inport  Port=2
  stiff_normal : Inport  Port=3
  stiff : Inport  Port=4
  Gain{1..6} (6 alike) : Gain  Gain=lamda
  Integrator{1..3,15} (4 alike) : Integrator
  Subtract{1..6,20..21} (8 alike) : Sum  Inputs=+-
  w_un_q_f : Outport
  dqq : Outport  Port=2
  w_un_s_f : Outport  Port=3
  dS : Outport  Port=4
  wires:
  w_q/1 -> Subtract20/1
  Subtract20/1 -> Gain2/1
  Subtract21/1 -> w_un_q_f/1
  Gain2/1 -> Integrator15/1
  Integrator15/1 -> Subtract21/2, Subtract20/2
  dq/1 -> Gain1/1
  Gain1/1 -> Subtract1/1, Subtract2/1
  Subtract1/1 -> Gain3/1
  Gain3/1 -> Integrator1/1
  Integrator1/1 -> Subtract1/2, Subtract2/2
  Subtract2/1 -> dqq/1, Subtract21/1
  Gain4/1 -> Integrator2/1
  Integrator2/1 -> w_un_s_f/1, Subtract3/2
  Subtract4/1 -> Subtract3/1
  Subtract3/1 -> Gain4/1
  stiff_normal/1 -> Subtract4/2
  Gain5/1 -> Subtract5/1, Subtract6/1
  Subtract6/1 -> dS/1
  Gain6/1 -> Integrator3/1
  Subtract5/1 -> Gain6/1
  Integrator3/1 -> Subtract5/2, Subtract6/2
  stiff/1 -> Subtract4/1

== matlab function CLNN_exp_3dof_2NN_exp/Theta error q ==
  data: Theta_q input; Theta_W_q input; Theta_error_q output; hat_W_vector_q input; hidden_neure_count_q input
function Theta_error_q  = fcn(Theta_q, Theta_W_q, hat_W_vector_q,hidden_neure_count_q)
% Theta_error = Theta_W - Theta * hat_W;

hidden_neure_count_q = 50; %40
output_dimension = 1*3;
hat_W_q = reshape(hat_W_vector_q,(hidden_neure_count_q + 1), output_dimension);
Theta_error_matrice_q = Theta_W_q - Theta_q * hat_W_q;

Theta_error_q = reshape(Theta_error_matrice_q,output_dimension*(hidden_neure_count_q + 1), 1);

== matlab function CLNN_exp_3dof_2NN_exp/MATLAB Function5 ==
  data: q input; activation output; theta1 input; theta2 input; activation_vec output; u1 input; u2 input
function [activation, activation_vec] = fcn(q, theta1, theta2, u1, u2)
activation = 1;
q1 = q(1:3);

activation_vec = [1,1,1];

for i = 1:3
    qi = q(i:i);
    theta1_i = theta1(i:i);
    theta2_i = theta2(i:i);
    u1_i = u1(i:i);
    u2_i = u2(i:i);

    if qi > 1.3
        activation = 0;
    end
    if qi <-1.3
         activation = 0;
    end
    
    if theta1_i > 2.5
        activation = 0;
    end
    if theta1_i <-2.5
         activation = 0;
    end
    
    if theta2_i > 2.5
        activation = 0;
    end
    if theta2_i <-2.5
         activation = 0;
    end

    if u1_i > 1.6
        activation = 0;
    end
    if u1_i <-1.6
         activation = 0;
    end

    if u2_i > 1.6
        activation = 0;
    end
    if u2_i <-1.6
         activation = 0;
    end
    

    activation_vec(:,i) = activation;
end

== matlab function CLNN_exp_3dof_2NN_exp/Subsystem4/qd2 ==
  data: t input; q output; q2 output; dq2 output; dqq2 output; dqqq2 output; dqqqq2 output; learn_time input
function [q,q2,dq2,dqq2,dqqq2,dqqqq2]  = fcn(t, learn_time)
%% exp q2

a  = 0;  %paper pi / 12
w = 0;   %paper 2
a1 = 1 * pi / 6; % paper pi / 6  paper pi / 6
w1 = pi / 8;    % paper pi /8     paper pi /8    

a = 0 * pi / 8;
w = pi / 9;

if t > learn_time
    % a1 = 1.0 * pi / 10;  %paper 1.0 * pi / 6;  
    % w1 = pi / 6;        %paper pi / 5;  
    a = 0 * pi / 8;
    w = pi / 6; 

    %20260510 task2 
    a1 = 0 * pi / 6; %
    w1 = pi / 8;    % 
end

% a1 = 0;
q = 16 *( a1 * sin(w1 * t) + 0*0.1 * pi + a * cos(w * t));  %paper 1*0.1 * pi


q2 = a * cos(w * t) - a + a1 * sin(w1 * t) + pi/2;
dq2 = -a * w * sin(w * t) + a1 * w1 * cos(w1 * t);
dqq2 = -a * w * w * cos(w * t) - a1 * w1 * w1 * sin(w1 * t);
dqqq2 = 0;
dqqqq2 = 0;
return;

== matlab function CLNN_exp_3dof_2NN_exp/THeta_WW_s/MATLAB Function ==
  data: u input; y output; t input; cl_tf1 input; cl_tf2 input
function y = fcn(u,t,cl_tf1, cl_tf2)
if t>cl_tf1 && t< cl_tf2
    y = u;
else
    y = zeros(31,3);  %31 x 3
end

== matlab function CLNN_exp_3dof_2NN_exp/w_un/MATLAB Function7 ==
  data: tau_e output; u1 input; u2 input; q input; theta1 input; theta2 input; M input; a1 input; kq1 input; a2 input; kq2 input; use_Tqr input; stiff output; stiff_normal output
function [tau_e, stiff, stiff_normal]  = fcn(u1, u2, q,theta1, theta2, M, a1, kq1, a2, kq2, use_Tqr)


q_theta1_real = q - theta1;
q_theta2_real = q - theta2;

q_theta1 = u1;
q_theta2 = u2;



%% plant stiffness
stiff = a1*kq1*cosh(a1*q_theta1_real) + a2*kq2*cosh(a2*q_theta2_real);


%% normal
tau_e = -2*q_theta1 - 2*q_theta2;
stiff_normal = 20*abs(q_theta1) + 30*abs(q_theta2);

== matlab function CLNN_exp_3dof_2NN_exp/MATLAB Function ==
  data: M input; w_q output; tau_e input; q input
function w_q = fcn(M, tau_e, q)

mgl2 = 0.45 * 9.8 *0.1;
% G_q = [0 G_q2 0]';
G_q = 0;
w_q = M^(-1) * (tau_e - G_q);

== matlab function CLNN_exp_3dof_2NN_exp/Subsystem4/qd3 ==
  data: t input; q output; q2 output; dq2 output; dqq2 output; dqqq2 output; dqqqq2 output; learn_time input
function [q,q2,dq2,dqq2,dqqq2,dqqqq2]  = fcn(t, learn_time)
%% exp 3

a  = 0;  %paper pi / 12
w = 0;   %paper 2


a1 = 1 * pi / 8; % paper pi / 6  paper pi / 6
w1 = pi / 6;    % paper pi /8     paper pi /8    

a = 0 * pi / 8;
w = pi / 9;

if t > learn_time
    % a1 = 1.0 * pi / 10;  %paper 1.0 * pi / 6;  
    % w1 = pi / 5;        %paper pi / 5;  
    a = 0 * pi / 8;
    w = pi / 6; 

    %20260510 task2 
    a1 = 0 * pi / 8; % 
    w1 = pi / 6;    %    
end


q = 16 *( a1 * sin(w1 * t) + 0*0.2 * pi); %16 *( a1 * sin(w1 * t) + 1*0.2 * pi); 


q2 = a * cos(w * t) - a + a1 * sin(w1 * t);
dq2 = -a * w * sin(w * t) + a1 * w1 * cos(w1 * t);
dqq2 = -a * w * w * cos(w * t) - a1 * w1 * w1 * sin(w1 * t);
dqqq2 = 0;
dqqqq2 = 0;
return;

== matlab function CLNN_exp_3dof_2NN_exp/THeta_WW_s/MATLAB Function Theta_W ==
  data: phi_filter_s input; phi_filter_W_s output; w_un_q_filter input; w_un_s_filter input
function phi_filter_W_s  = fcn(phi_filter_s,  w_un_q_filter, w_un_s_filter)
% w_un_filter = [w_un_q_filter; w_un_s_filter];
phi_filter_W_s = phi_filter_s * w_un_s_filter';

== matlab function CLNN_exp_3dof_2NN_exp/Theta_s/MATLAB Function ==
  data: u input; y output; t input; cl_tf1 input; cl_tf2 input
function y = fcn(u,t,cl_tf1, cl_tf2)
if t>cl_tf1 && t< cl_tf2
    y = u;
else
    y = zeros(31,31); %31 * 31
end

== matlab function CLNN_exp_3dof_2NN_exp/Theta_s/MATLAB Function Theta ==
  data: phi_filter input; phi_filter_phi_filter output; hidden_neure_count input
function phi_filter_phi_filter  = fcn(phi_filter,hidden_neure_count)
phi_filter_phi_filter_m = phi_filter * phi_filter';
% temp = zeros(hidden_neure_count*hidden_neure_count,1);
% phi_filter_phi_filter = zeros(625*625);
% for i =1:hidden_neure_count
%     for j = 1:hidden_neure_count
%         temp((i-1)*hidden_neure_count + j) = phi_filter_phi_filter_m(i,j);
%     end
% end
phi_filter_phi_filter = phi_filter_phi_filter_m;
% phi_filter_phi_filter = zeros(625,625);

== matlab function CLNN_exp_3dof_2NN_exp/Theta error s ==
  data: Theta_s input; Theta_W_s input; Theta_error_s output; hat_W_vector_s input; hidden_neure_count_s input
function Theta_error_s  = fcn(Theta_s, Theta_W_s, hat_W_vector_s, hidden_neure_count_s)
% Theta_error = Theta_W - Theta * hat_W;

hidden_neure_count_s = 30; %30
output_dimension = 1*3;
hat_W_s = reshape(hat_W_vector_s,(hidden_neure_count_s + 1), output_dimension);
Theta_error_matrice_s = Theta_W_s - Theta_s * hat_W_s;

Theta_error_s = reshape(Theta_error_matrice_s,output_dimension*(hidden_neure_count_s + 1), 1);

== matlab function CLNN_exp_3dof_2NN_exp/stiff and tau1/stiffness ==
  data: tau_e output; theta1 input; theta2 input; q input; a1 input; kq1 input; a2 input; kq2 input; stiffness output
function [tau_e, stiffness ] = fcn(theta1, theta2, q, a1, kq1, a2, kq2)


q_theta1 = q - theta1;
q_theta2 = q - theta2;

tau_e =  -kq1 * sinh(a1*q_theta1) - kq2 * sinh(a2*q_theta2);

stiffness = a1 * kq1 * cosh(a1*q_theta1) + a2 * kq2 * cosh(a2*q_theta2);

== matlab function CLNN_exp_3dof_2NN_exp/Theta_q/MATLAB Function ==
  data: u input; y output; t input; cl_tf1 input; cl_tf2 input
function y = fcn(u,t,cl_tf1, cl_tf2)
if t>cl_tf1 && t< cl_tf2
    y = u;
else
    y = zeros(51, 51); %N_q = 41
end

== matlab function CLNN_exp_3dof_2NN_exp/Subsystem4/qd1 ==
  data: t input; q output; q2 output; dq2 output; dqq2 output; dqqq2 output; dqqqq2 output; learn_time input
function [q,q2,dq2,dqq2,dqqq2,dqqqq2]  = fcn(t, learn_time)

%% exp q1


%%%%cos  
a  = 0;  %paper pi / 12
w = 0;   %paper 2

a1 = 1 * pi / 5; % paper  pi / 5  paper  pi / 4
w1 = pi / 10;   % paper pi /10    paper pi /10

a = 0 * pi / 8;
w = pi / 8;

if t > learn_time
    a1 = 1.0 * pi / 8;  %paper 1.0 * pi / 6
    w1 = pi / 8;         %paper  pi / 6

    a = 0 * pi / 8;
    w = pi / 10;

    %20260510 task2 
    a1 = 0 * pi / 5; % 
    w1 = pi / 10;   % 
end

q = 16 *( a1 * sin(w1 * t) + 0*0.1 * pi + a * cos(w * t)); % paper 1*0.2 * pi



q2 = a * cos(w * t) - a + a1 * sin(w1 * t);
dq2 = -a * w * sin(w * t) + a1 * w1 * cos(w1 * t);
dqq2 = -a * w * w * cos(w * t) - a1 * w1 * w1 * sin(w1 * t);
dqqq2 = 0;
dqqqq2 = 0;
return;

== matlab function CLNN_exp_3dof_2NN_exp/s/sd1 ==
  data: t input; q output; q2 output; dq2 output; dqq2 output; dqqq2 output; dqqqq2 output; learn_time input
function [q,q2,dq2,dqq2,dqqq2,dqqqq2]  = fcn(t, learn_time)

%% exp s1

a  = 0;  %paper pi / 12
w = 0;   %paper 2

%stiffness baseline
a_s = 8;

a1 = 1.8 * pi / 1; %  paper 1.8 * pi / 1 
w1 = pi / 10;        % paper pi / 10    

if t> learn_time
    a1 = 1.2 * pi / 1; %paper 1.2 * pi / 1
    w1 = pi / 8;        % paper pi / 8  

    a1 = 0;
    a_s = 4;
end

q = 16 *( a1 * sin(w1 * t) + 1* a_s * pi);  %paper 1* 8 * pi


q2 = a * cos(w * t) - a + a1 * sin(w1 * t);
dq2 = -a * w * sin(w * t) + a1 * w1 * cos(w1 * t);
dqq2 = -a * w * w * cos(w * t) - a1 * w1 * w1 * sin(w1 * t);
dqqq2 = 0;
dqqqq2 = 0;
return;

== matlab function CLNN_exp_3dof_2NN_exp/s/sd2 ==
  data: t input; q output; q2 output; dq2 output; dqq2 output; dqqq2 output; dqqqq2 output; learn_time input
function [q,q2,dq2,dqq2,dqqq2,dqqqq2]  = fcn(t, learn_time)
%% exp s2
a  = 0;  %paper pi / 12
w = 0;   %paper 2

a1 = 0.8 * pi / 1; % paper 0.8 * pi / 1;  
w1 = pi / 10;   % paper pi /10

%stiffness baseline
a_s = 6;

if t> learn_time
    a1 = 0.5 * pi / 1; %paper 0.8 * pi / 1
    w1 = pi / 8;        % paper pi / 6  

    a1 = 0;   %6
    a_s = 1;
end

q = 16 *( a1 * sin(w1 * t) + 1* a_s * pi);   % paper 1*6 * pi

q2 = a * cos(w * t) - a + a1 * sin(w1 * t) + pi/2;
dq2 = -a * w * sin(w * t) + a1 * w1 * cos(w1 * t);
dqq2 = -a * w * w * cos(w * t) - a1 * w1 * w1 * sin(w1 * t);
dqqq2 = 0;
dqqqq2 = 0;
return;

== matlab function CLNN_exp_3dof_2NN_exp/s/sd3 ==
  data: t input; q output; q2 output; dq2 output; dqq2 output; dqqq2 output; dqqqq2 output; learn_time input
function [q,q2,dq2,dqq2,dqqq2,dqqqq2]  = fcn(t, learn_time)
%% exp s3
a  = 0;  %paper pi / 12
w = 0;   %paper 2

a1 = 1 * pi / 1; % paper 0.8 * pi / 1;  
w1 = pi / 8;   % paper pi /10   

%stiffness baseline
a_s = 5;

if t> learn_time
    a1 = 0.5 * pi / 1; %paper 0.8 * pi / 1
    w1 = pi / 8;        % paper pi / 6  

    a1 = 0;
    a_s = 3;
end

q = 16 *( a1 * sin(w1 * t) + 1* a_s * pi);   % paper 1*5 * pi

q2 = a * cos(w * t) - a + a1 * sin(w1 * t);
dq2 = -a * w * sin(w * t) + a1 * w1 * cos(w1 * t);
dqq2 = -a * w * w * cos(w * t) - a1 * w1 * w1 * sin(w1 * t);
dqqq2 = 0;
dqqqq2 = 0;
return;

== matlab function CLNN_exp_3dof_2NN_exp/Theta_q/MATLAB Function Theta ==
  data: phi_filter_q input; phi_filter_phi_filter_q output; hidden_neure_count_q input
function phi_filter_phi_filter_q  = fcn(phi_filter_q,hidden_neure_count_q)
phi_filter_phi_filter_m = phi_filter_q * phi_filter_q';

phi_filter_phi_filter_q = phi_filter_phi_filter_m;
% phi_filter_phi_filter = zeros(625,625);

== matlab function CLNN_exp_3dof_2NN_exp/THeta_WW_q/MATLAB Function Theta_W ==
  data: phi_filter_q input; phi_filter_W_q output; w_un_q_filter input; w_un_s_filter input
function phi_filter_W_q  = fcn(phi_filter_q,  w_un_q_filter, w_un_s_filter)
% w_un_filter = [w_un_q_filter; w_un_s_filter];
phi_filter_W_q = phi_filter_q * w_un_q_filter';

== matlab function CLNN_exp_3dof_2NN_exp/THeta_WW_q/MATLAB Function ==
  data: u input; y output; t input; cl_tf1 input; cl_tf2 input
function y = fcn(u,t,cl_tf1, cl_tf2)
if t>cl_tf1 && t< cl_tf2
    y = u;
else
    y = zeros(51,3);  %41 x 6
end

== matlab function CLNN_exp_3dof_2NN_exp/MATLAB Function6 ==
  data: output input; w_un_hat output; epsion output; w_norm_q output; w_norm_s output; controlu1 output; controlu2 output; u_theta1 output; u_theta2 output; pd_u output; model_u output; W_q output; hidden_neure_count_q input; hidden_neure_count_s input; N input; q input; W_s output
function [w_un_hat, epsion, w_norm_q,w_norm_s,controlu1, controlu2, u_theta1, u_theta2,pd_u, model_u, W_q, W_s] = fcn(output, hidden_neure_count_q,hidden_neure_count_s,N,q)
N = 3;
output_dimension = 2*N;

w_un_hat = output(1:output_dimension);
epsion =  output((output_dimension + 1):(2 * output_dimension));
controlu1 = output((2 * output_dimension +1):(2 * output_dimension + N));
controlu2 = output((2 * output_dimension + N +1):(2 * output_dimension + 2 * N));

pd_u = 0;
model_u = 0;
u_theta1 = q - controlu1;
u_theta2 = q - controlu2;


hidden_neure_count_q = 50; %40
hidden_neure_count_s = 30; %30
N_wq = N *(hidden_neure_count_q +1);
N_ws = N *(hidden_neure_count_s +1);

w_norm_temp_q = 0;
for i = (2 * output_dimension + 2 * N + 1):(N_wq + 2 * output_dimension + 2 * N)
    w_norm_temp_q = w_norm_temp_q + output(i) * output(i);
end
w_norm_q = w_norm_temp_q;

w_norm_temp_s = 0;
for i = (N_wq + 2 * output_dimension + 2 * N + 1):(N_wq + N_ws + 2 * output_dimension + 2 * N)
    w_norm_temp_s = w_norm_temp_s + output(i) * output(i);
end
w_norm_s = w_norm_temp_s;

W_q = output((2 * output_dimension + 2 * N + 1):(2 * output_dimension + 2 * N + N_wq));
W_s = output((2 * output_dimension + 2 * N + N_wq + 1):end);
